simulink model "pvcells"  (R2024a)
settings: Solver=VariableStepAuto  StartTime=0.0  StopTime=40  RelTol=1e-3
undefined symbols (not defined in the file): e, isc, k, ki, n, ns, q, rs, rsh, tn, voc
libraries: simulink x1
settings Model: Creator=RAMANJANEYULU  LastModifiedBy=RAMANJANEYULU
settings DebuggingCC: AlgebraicLoopMsg=none  ArtificialAlgebraicLoopMsg=none

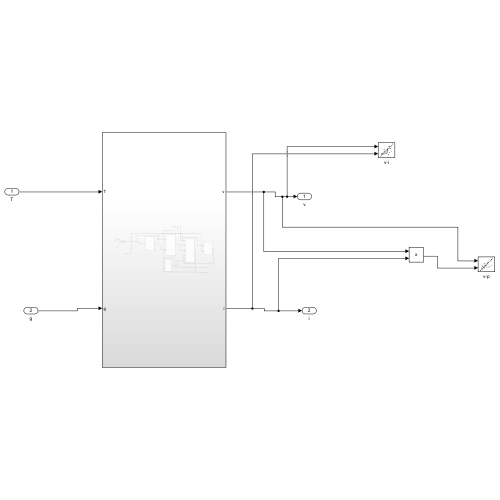
[thumbnail: Simulink's stored preview of the top-level diagram]
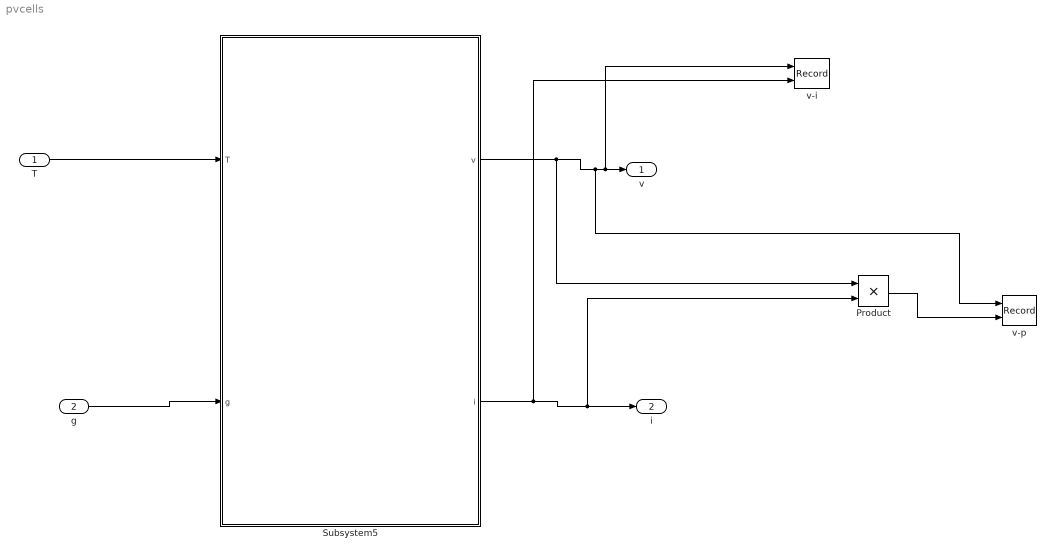
== system pvcells ==
  T : Inport
  g : Inport  Port=2
  Product : Product
  Subsystem5 : Subsystem
  v-i : Record  FileSettingsInternal="{\"entries\":[{\"content\":{\"excelSettings\":{\"content\":{},\"type\":\"Streamout.ExcelSettings\"}},\"type\":\"Streamout.FileSettingStorage\",\"uuid\":\"\"}],\"packageUris\":[\"http:\\/\\/schema.mathworks.com\\/mf0\\/streamout_blocks\\/R2020a\"],\"version\":\"1.0\"}"  Layout=[1 1]  SignalsInternal="{\"entries\":[{\"content\":{\"signals\":[{\"content\":{\"blockPath\":[],\"dimensions\":[1],\"domain\":\"\",\"lineColor\":\"#a2142f\",\"plots\":[ 1 ],\"port\":1,\"sid\":[\"\"],\"signalID\":1,\"signalName\":\"Subsystem5:1\"},\"type\":\"RecordBlkView.Signal\",\"uuid\":\"\"},{\"content\":{\"blockPath\":[],\"dimensions\":[1],\"domain\":\"\",\"lineColor\":\"#139fff\",\"plots\":[ 1 ],\"port\":2,\"sid\":[\"\"],\"signalID\":2,\"signalName\":\"Subsystem5:2\"},\"type\":\"RecordBlkView.Signal\",\"uuid\":\"\"}]},\"type\":\"RecordBlkView.InputSignals\",\"uuid\":\"\"}],\"packageUris\":[\"http:\\/\\/schema.mathworks.com\\/mf0\\/streamout_blocks\\/R2020a\"],\"version\":\"1.0\"}"  VisualizationBindings="{\"xyplotplugin\":{\"info\":[{\"series\":[{\"bindingParametersList\":[{\"parameter\":\"X-Axis\",\"signalID\":1,\"signalName\":\"Subsystem5:1\"},{\"parameter\":\"Y-Axis\",\"signalID\":2,\"signalName\":\"Subsystem5:2\"}],\"seriesID\":0}],\"subplotID\":1}]}}"  CompatibilityTag=XY
  v-p : Record  FileSettingsInternal="{\"entries\":[{\"content\":{\"excelSettings\":{\"content\":{},\"type\":\"Streamout.ExcelSettings\"}},\"type\":\"Streamout.FileSettingStorage\",\"uuid\":\"\"}],\"packageUris\":[\"http:\\/\\/schema.mathworks.com\\/mf0\\/streamout_blocks\\/R2020a\"],\"version\":\"1.0\"}"  Layout=[1 1]  SignalsInternal="{\"entries\":[{\"content\":{\"signals\":[{\"content\":{\"blockPath\":[],\"dimensions\":[1],\"domain\":\"\",\"lineColor\":\"#a2142f\",\"plots\":[ 1 ],\"port\":1,\"sid\":[\"\"],\"signalID\":1,\"signalName\":\"Subsystem5:1\"},\"type\":\"RecordBlkView.Signal\",\"uuid\":\"\"},{\"content\":{\"blockPath\":[],\"dimensions\":[1],\"domain\":\"\",\"lineColor\":\"#139fff\",\"plots\":[ 1 ],\"port\":2,\"sid\":[\"\"],\"signalID\":2,\"signalName\":\"Product\"},\"type\":\"RecordBlkView.Signal\",\"uuid\":\"\"}]},\"type\":\"RecordBlkView.InputSignals\",\"uuid\":\"\"}],\"packageUris\":[\"http:\\/\\/schema.mathworks.com\\/mf0\\/streamout_blocks\\/R2020a\"],\"version\":\"1.0\"}"  VisualizationBindings="{\"xyplotplugin\":{\"info\":[{\"series\":[{\"bindingParametersList\":[{\"parameter\":\"X-Axis\",\"signalID\":1,\"signalName\":\"Subsystem5:1\"},{\"parameter\":\"Y-Axis\",\"signalID\":2,\"signalName\":\"Product\"}],\"seriesID\":0}],\"subplotID\":1}]}}"  CompatibilityTag=XY
  v : Outport
  i : Outport  Port=2
  wires:
  T/1 -> Subsystem5/1(T)
  g/1 -> Subsystem5/2(g)
  Subsystem5/2(i) -> v-i/2, Product/2, i/1
  Product/1 -> v-p/2
  Subsystem5/1(v) -> Product/1, v-p/1, v-i/1, v/1

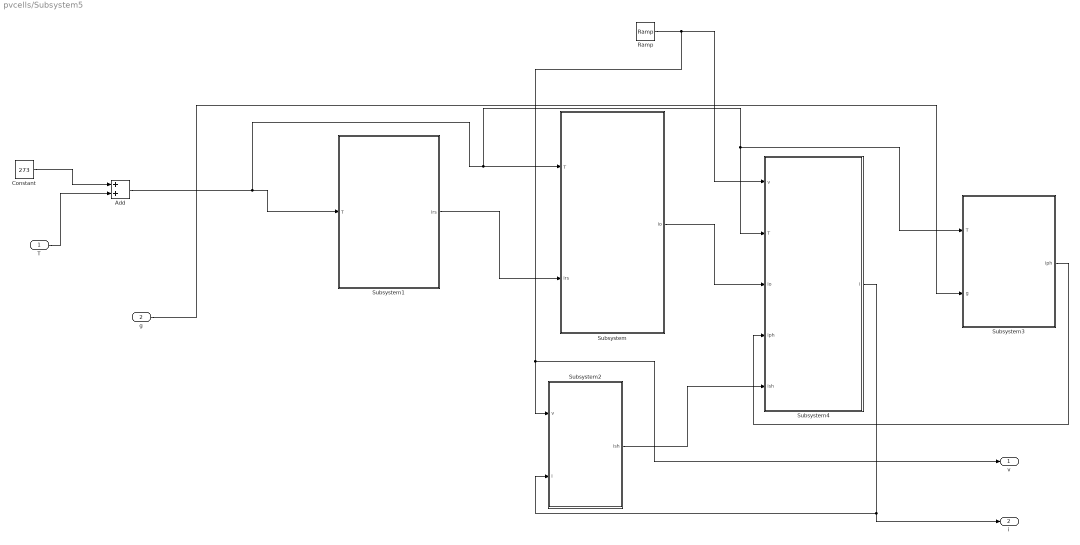
== system pvcells/Subsystem5 ==
  T : Inport
  g : Inport  Port=2
  Add : Sum
  Constant : Constant  Value=273
  Ramp : simulink/Sources/Ramp  slope=1  start=0  InitialOutput=0
  Subsystem : Subsystem
  Subsystem1 : Subsystem
  Subsystem2 : Subsystem
  Subsystem3 : Subsystem
  Subsystem4 : Subsystem
  v : Outport
  i : Outport  Port=2
  wires:
  Subsystem1/1(irs) -> Subsystem/2(irs)
  Subsystem/1(io) -> Subsystem4/3(io)
  Ramp/1 -> v/1, Subsystem2/1(v), Subsystem4/1(v)
  Subsystem3/1(iph) -> Subsystem4/4(iph)
  Subsystem2/1(ish) -> Subsystem4/5(ish)
  Subsystem4/1(i) -> i/1, Subsystem2/2(i)
  g/1 -> Subsystem3/2(g)
  Constant/1 -> Add/1
  T/1 -> Add/2
  Add/1 -> Subsystem3/1(T), Subsystem4/2(T), Subsystem/1(T), Subsystem1/1(T)

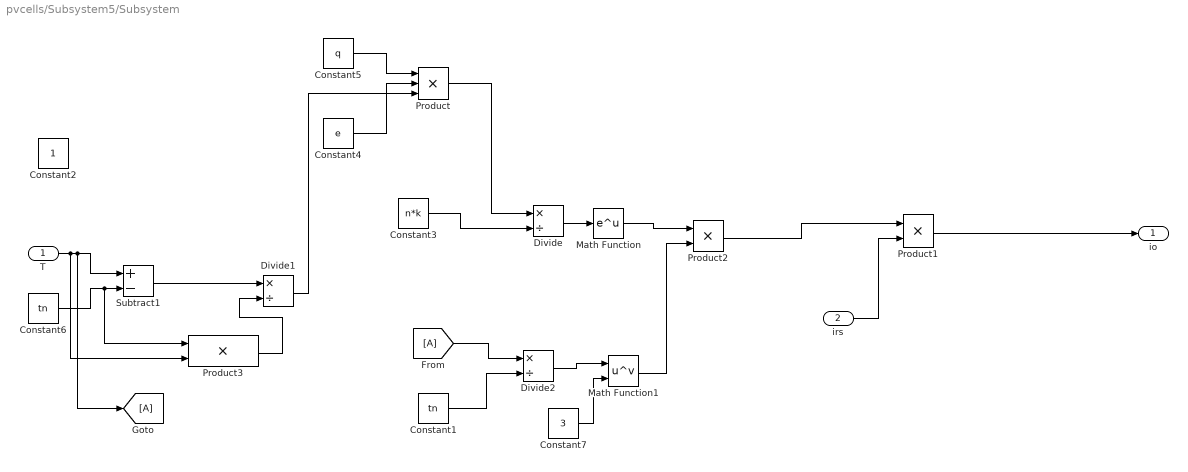
== system pvcells/Subsystem5/Subsystem ==
  T : Inport
  irs : Inport  Port=2
  Constant1 : Constant  Value=tn
  Constant2 : Constant
  Constant3 : Constant  Value=n*k
  Constant4 : Constant  Value=e
  Constant5 : Constant  Value=q
  Constant6 : Constant  Value=tn
  Constant7 : Constant  Value=3
  Divide : Product  Inputs=*/
  Divide1 : Product  Inputs=*/
  Divide2 : Product  Inputs=*/
  From : From
  Goto : Goto
  Math Function : Math
  Math Function1 : Math  Operator=pow
  Product : Product  Inputs=3
  Product1 : Product
  Product2 : Product
  Product3 : Product
  Subtract1 : Sum  Inputs=+-
  io : Outport
  wires:
  Product/1 -> Divide/1
  Constant5/1 -> Product/1
  Constant4/1 -> Product/2
  Constant3/1 -> Divide/2
  irs/1 -> Product1/2
  Product1/1 -> io/1
  Divide/1 -> Math Function/1
  Math Function/1 -> Product2/1
  From/1 -> Divide2/1
  Constant1/1 -> Divide2/2
  Divide2/1 -> Math Function1/1
  Constant7/1 -> Math Function1/2
  Math Function1/1 -> Product2/2
  Product2/1 -> Product1/1
  T/1 -> Product3/2, Goto/1, Subtract1/1
  Constant6/1 -> Product3/1, Subtract1/2
  Subtract1/1 -> Divide1/1
  Product3/1 -> Divide1/2
  Divide1/1 -> Product/3

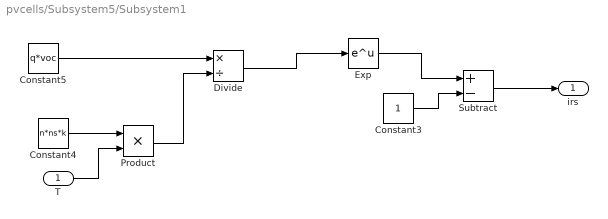
== system pvcells/Subsystem5/Subsystem1 ==
  T : Inport
  Constant3 : Constant
  Constant4 : Constant  Value=n*ns*k
  Constant5 : Constant  Value=q*voc
  Divide : Product  Inputs=*/
  Exp : Math  SignedPower=on
  Product : Product
  Subtract : Sum  Inputs=+-
  irs : Outport
  wires:
  Subtract/1 -> irs/1
  Constant3/1 -> Subtract/2
  T/1 -> Product/2
  Product/1 -> Divide/2
  Constant4/1 -> Product/1
  Exp/1 -> Subtract/1
  Constant5/1 -> Divide/1
  Divide/1 -> Exp/1

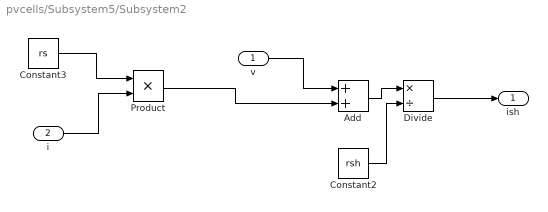
== system pvcells/Subsystem5/Subsystem2 ==
  v : Inport
  i : Inport  Port=2
  Add : Sum
  Constant2 : Constant  Value=rsh
  Constant3 : Constant  Value=rs
  Divide : Product  Inputs=*/
  Product : Product
  ish : Outport
  wires:
  Product/1 -> Add/2
  Constant2/1 -> Divide/2
  v/1 -> Add/1
  Add/1 -> Divide/1
  Constant3/1 -> Product/1
  i/1 -> Product/2
  Divide/1 -> ish/1

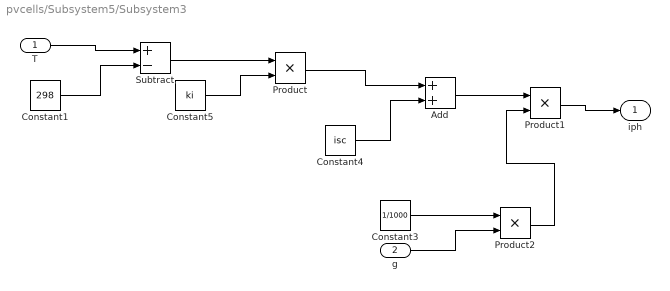
== system pvcells/Subsystem5/Subsystem3 ==
  T : Inport
  g : Inport  Port=2
  Add : Sum
  Constant1 : Constant  Value=298
  Constant3 : Constant  Value=1/1000
  Constant4 : Constant  Value=isc
  Constant5 : Constant  Value=ki
  Product : Product
  Product1 : Product
  Product2 : Product
  Subtract : Sum  Inputs=+-
  iph : Outport
  wires:
  Subtract/1 -> Product/1
  Constant4/1 -> Add/2
  Add/1 -> Product1/1
  Constant1/1 -> Subtract/2
  Constant5/1 -> Product/2
  T/1 -> Subtract/1
  Product/1 -> Add/1
  Constant3/1 -> Product2/1
  g/1 -> Product2/2
  Product2/1 -> Product1/2
  Product1/1 -> iph/1

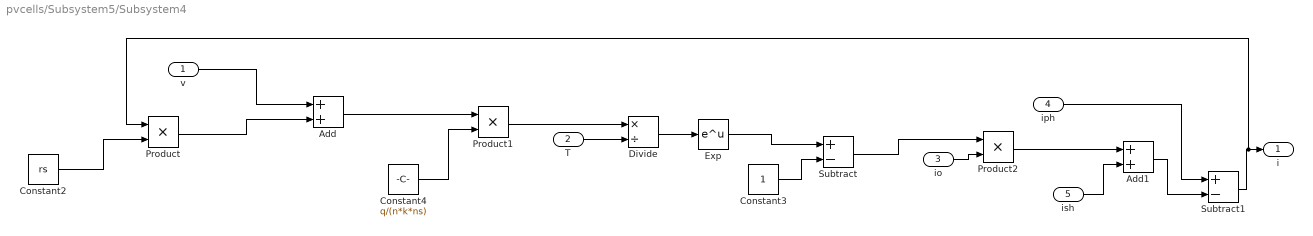
== system pvcells/Subsystem5/Subsystem4 ==
  v : Inport
  T : Inport  Port=2
  io : Inport  Port=3
  iph : Inport  Port=4
  ish : Inport  Port=5
  Add : Sum
  Add1 : Sum
  Constant2 : Constant  Value=rs
  Constant3 : Constant
  Constant4 : Constant  Value=q/(n*k*ns)
  Divide : Product  Inputs=*/
  Exp : Math
  Product : Product
  Product1 : Product
  Product2 : Product
  Subtract : Sum  Inputs=+-
  Subtract1 : Sum  Inputs=+-
  i : Outport
  wires:
  v/1 -> Add/1
  Subtract/1 -> Product2/1
  Product2/1 -> Add1/1
  Constant3/1 -> Subtract/2
  Product/1 -> Add/2
  Exp/1 -> Subtract/1
  Constant4/1 -> Product1/2
  Divide/1 -> Exp/1
  io/1 -> Product2/2
  Add/1 -> Product1/1
  Constant2/1 -> Product/2
  Product1/1 -> Divide/1
  T/1 -> Divide/2
  ish/1 -> Add1/2
  iph/1 -> Subtract1/1
  Add1/1 -> Subtract1/2
  Subtract1/1 -> Product/1, i/1
